simulink model "Power_meter_All_Watts"  (R2022a)
settings: Solver=VariableStepAuto  StartTime=0.0  StopTime=3  RelTol=1e-3
libraries: dspstat3 x1, dspsrcs4 x1
settings Model: Creator=EVSHI2  LastModifiedBy=EVSHI2
settings DataIOCC: ReturnWorkspaceOutputs=off

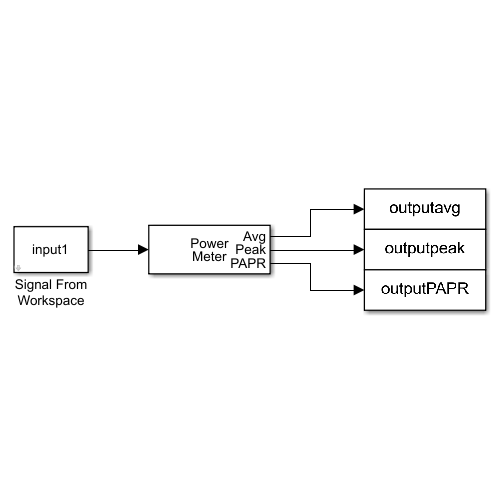
[thumbnail: Simulink's stored preview of the top-level diagram]
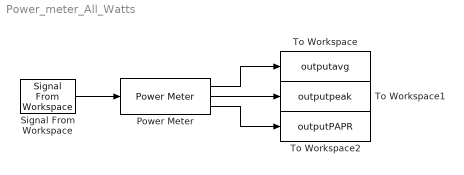
== system Power_meter_All_Watts ==
  Power Meter : dspstat3/Power Meter  Measurement=All  WindowLength=4  ReferenceLoad=1  OutputPowerUnits=Watts  SimulateUsing=Code generation
      settings: SourceProductBaseCode=DS
  Signal From Workspace : dspsrcs4/Signal From Workspace  X=input1  Ts=1  nsamps=1  OutputAfterFinalValue=Setting to zero  ignoreOrWarnInputAndFrameLengths=off  OutputFrames=off
  To Workspace : ToWorkspace  VariableName=outputavg  SampleTime=-1
      settings: Save2DSignal=2-D array (concatenate along first dimension)
  To Workspace1 : ToWorkspace  VariableName=outputpeak  SampleTime=-1
      settings: Save2DSignal=2-D array (concatenate along first dimension)
  To Workspace2 : ToWorkspace  VariableName=outputPAPR  SampleTime=-1
      settings: Save2DSignal=2-D array (concatenate along first dimension)
  wires:
  Power Meter/1 -> To Workspace/1
  Signal From Workspace/1 -> Power Meter/1
  Power Meter/2 -> To Workspace1/1
  Power Meter/3 -> To Workspace2/1
